simulink model "ADU_Integration_Y2016_simulation"  (R2016b)
settings: Solver=FixedStepDiscrete  StartTime=240  StopTime=300  FixedStep=0.01  RelTol=1e-3  EnableMultiTasking=on
PostLoadFcn:
  | , if any(exist('dsrtsu_mdlpostloadfcn', 'file') == [2, 3, 6]), try dsrtsu_mdlpostloadfcn('Execute', bdroot); catch fprintf('Error in PostLoadFcn (dsrtsu_mdlpostloadfcn) for model "%s":\n %s\n', bdroot, lasterr); end, end,
InitFcn:
  | load 'data/chi2_dat';
  | load 'data/innerLine_struct';
  | load 'data/middleLine_struct';
  | load 'data/outerLine_struct';
  | load 'data/innerLine';
  | load 'data/middleLine';
  | load 'data/outerLine';
  | load 'data/landmarks_patac_schimmel_ccw';
  | load 'data/patac_navi_array';
  | load 'data/sensor';
  | load 'data/map_struct';
  | addpath map_src
  | Integration_Parameter;
  | load 'TestData_001';
values from neighbouring files (symbols this model uses):
  TestData_001 =     [TestData_001.mat]
undefined symbols (not defined in the file or in its folder): a, chi2_dat, innerLine, landmarks_patac_schimmel_ccw, middleLine, outerLine, patac_navi_array, StartNum
libraries: simulink x36, rtican x1
(part 7 of 20)

== system ADU_Integration_Y2016_simulation/LogData/Vision_Target/EPM_Lane_Signals ==
  1-D Lookup Table1 : Lookup_n-D  NumberOfTableDimensions=1  BreakpointsForDimension1=TestData_001.X.Data  Table=TestData_001.Y(667).Data  RndMeth=Simplest  InputSameDT=on
  1-D Lookup Table10 : Lookup_n-D  NumberOfTableDimensions=1  BreakpointsForDimension1=TestData_001.X.Data  Table=TestData_001.Y(687).Data  RndMeth=Simplest  InputSameDT=on
  1-D Lookup Table11 : Lookup_n-D  NumberOfTableDimensions=1  BreakpointsForDimension1=TestData_001.X.Data  Table=TestData_001.Y(688).Data  RndMeth=Simplest  InputSameDT=on
  1-D Lookup Table12 : Lookup_n-D  NumberOfTableDimensions=1  BreakpointsForDimension1=TestData_001.X.Data  Table=TestData_001.Y(689).Data  RndMeth=Simplest  InputSameDT=on
  1-D Lookup Table13 : Lookup_n-D  NumberOfTableDimensions=1  BreakpointsForDimension1=TestData_001.X.Data  Table=TestData_001.Y(692).Data  RndMeth=Simplest  InputSameDT=on
  1-D Lookup Table14 : Lookup_n-D  NumberOfTableDimensions=1  BreakpointsForDimension1=TestData_001.X.Data  Table=TestData_001.Y(694).Data  RndMeth=Simplest  InputSameDT=on
  1-D Lookup Table15 : Lookup_n-D  NumberOfTableDimensions=1  BreakpointsForDimension1=TestData_001.X.Data  Table=TestData_001.Y(695).Data  RndMeth=Simplest  InputSameDT=on
  1-D Lookup Table190 : Lookup_n-D  NumberOfTableDimensions=1  BreakpointsForDimension1=TestData_001.X.Data  Table=TestData_001.Y(666).Data  RndMeth=Simplest  InputSameDT=on
  1-D Lookup Table2 : Lookup_n-D  NumberOfTableDimensions=1  BreakpointsForDimension1=TestData_001.X.Data  Table=TestData_001.Y(663).Data  RndMeth=Simplest  InputSameDT=on
  1-D Lookup Table3 : Lookup_n-D  NumberOfTableDimensions=1  BreakpointsForDimension1=TestData_001.X.Data  Table=TestData_001.Y(664).Data  RndMeth=Simplest  InputSameDT=on
  1-D Lookup Table4 : Lookup_n-D  NumberOfTableDimensions=1  BreakpointsForDimension1=TestData_001.X.Data  Table=TestData_001.Y(665).Data  RndMeth=Simplest  InputSameDT=on
  1-D Lookup Table5 : Lookup_n-D  NumberOfTableDimensions=1  BreakpointsForDimension1=TestData_001.X.Data  Table=TestData_001.Y(668).Data  RndMeth=Simplest  InputSameDT=on
  1-D Lookup Table6 : Lookup_n-D  NumberOfTableDimensions=1  BreakpointsForDimension1=TestData_001.X.Data  Table=TestData_001.Y(670).Data  RndMeth=Simplest  InputSameDT=on
  1-D Lookup Table7 : Lookup_n-D  NumberOfTableDimensions=1  BreakpointsForDimension1=TestData_001.X.Data  Table=TestData_001.Y(671).Data  RndMeth=Simplest  InputSameDT=on
  1-D Lookup Table8 : Lookup_n-D  NumberOfTableDimensions=1  BreakpointsForDimension1=TestData_001.X.Data  Table=TestData_001.Y(690).Data  RndMeth=Simplest  InputSameDT=on
  1-D Lookup Table9 : Lookup_n-D  NumberOfTableDimensions=1  BreakpointsForDimension1=TestData_001.X.Data  Table=TestData_001.Y(691).Data  RndMeth=Simplest  InputSameDT=on
  Bus Creator{,3,5,7} (4 alike) : BusCreator  Inputs=7
  Bus Creator1 : BusCreator  Inputs=19
  Bus Creator2 : BusCreator  Inputs=8
  Bus Creator4 : BusCreator  Inputs=19
  Bus Creator6 : BusCreator  Inputs=6
  Bus Creator8 : BusCreator  Inputs=6
  EPM_Lane_Singals : Outport
  wires:
  Bus Creator/1 -> Bus Creator2/1  "LKA_Left_Lane_A"
  ? -> Bus Creator3/7  "Rx_Time"
  Bus Creator2/1 -> EPM_Lane_Singals/1  "EPM_Lane_BUS"
  Bus Creator3/1 -> Bus Creator2/3  "LKA_Right_Lane_A"
  1-D Lookup Table8/1 -> Bus Creator3/1  "Lane_Type"
  1-D Lookup Table9/1 -> Bus Creator3/2  "Quality"
  Bus Creator4/1 -> Bus Creator2/4  "LKA_Right_Lane_B"
  Bus Creator1/1 -> Bus Creator2/2  "LKA_Left_Lane_B"
  1-D Lookup Table1/1 -> Bus Creator/2  "Quality"
  1-D Lookup Table190/1 -> Bus Creator/1  "Lane_Type"
  ? -> Bus Creator5/2  "Quality"
  ? -> Bus Creator5/1  "Lane_Type"
  ? -> Bus Creator5/7  "Rx_Time"
  ? -> Bus Creator7/2  "Quality"
  ? -> Bus Creator7/1  "Lane_Type"
  ? -> Bus Creator7/7  "Rx_Time"
  Bus Creator8/1 -> Bus Creator2/8  "Next_Right_Lane_B"
  Bus Creator7/1 -> Bus Creator2/7  "Next_Right_Lane_A"
  Bus Creator5/1 -> Bus Creator2/5  "Next_Left_Lane_A"
  Bus Creator6/1 -> Bus Creator2/6  "Next_Left_Lane_B"
  1-D Lookup Table4/1 -> Bus Creator/5  "Lane_Model_C3"
  1-D Lookup Table2/1 -> Bus Creator/3  "Lane_Model_C0"
  1-D Lookup Table5/1 -> Bus Creator/6  "Width_marking"
  1-D Lookup Table3/1 -> Bus Creator/4  "Lane_Model_C2"
  1-D Lookup Table6/1 -> Bus Creator1/1  "Lane_Model_C1"
  ? -> Bus Creator1/4  "reserved2_laneB"
  ? -> Bus Creator1/18  "TLC"
  ? -> Bus Creator1/9  "PRED_OVERRIDE"
  ? -> Bus Creator1/12  "Reserved1_laneB"
  ? -> Bus Creator1/2  "View_Range_Start"
  ? -> Bus Creator1/16  "PRED_SOURCE_STD"
  ? -> Bus Creator1/15  "PRED_SOURCE_HWE_SPAIN"
  ? -> Bus Creator1/5  "Lane_Crossing"
  1-D Lookup Table7/1 -> Bus Creator1/6  "Lane_mark_color"
  ? -> Bus Creator1/7  "PRED_DIST_BASED_EXTRAPOLATION"
  ? -> Bus Creator1/10  "PRED_OCCLUDED_LM_EXTRAPOLATION"
  ? -> Bus Creator1/11  "PRED_HEADWAY_ORIENTED"
  ? -> Bus Creator1/13  "PRED_SOURCE_DIVERGING_LANES"
  ? -> Bus Creator1/14  "PRED_SOURCE_GUARDRAIL_SHADOW"
  ? -> Bus Creator1/17  "PRED_SOURCE_VRTL_MERGE"
  ? -> Bus Creator1/19  "Rx_Time"
  ? -> Bus Creator1/3  "View_Range_End"
  ? -> Bus Creator1/8  "PRED_OTHER_SIDE"
  1-D Lookup Table12/1 -> Bus Creator3/5  "Lane_Model_C3"
  1-D Lookup Table13/1 -> Bus Creator3/6  "Width_marking"
  1-D Lookup Table10/1 -> Bus Creator3/3  "Lane_Model_C0"
  1-D Lookup Table11/1 -> Bus Creator3/4  "Lane_Model_C2"
  1-D Lookup Table14/1 -> Bus Creator4/1  "Lane_Model_C1"
  ? -> Bus Creator4/3  "View_Range_End"
  ? -> Bus Creator4/10  "PRED_OCCLUDED_LM_EXTRAPOLATION"
  ? -> Bus Creator4/12  "Reserved1_laneB"
  ? -> Bus Creator4/14  "PRED_SOURCE_GUARDRAIL_SHADOW"
  ? -> Bus Creator4/2  "View_Range_Start"
  ? -> Bus Creator4/5  "Lane_Crossing"
  1-D Lookup Table15/1 -> Bus Creator4/6  "Lane_mark_color"
  ? -> Bus Creator4/7  "PRED_DIST_BASED_EXTRAPOLATION"
  ? -> Bus Creator4/8  "PRED_OTHER_SIDE"
  ? -> Bus Creator4/11  "PRED_HEADWAY_ORIENTED"
  ? -> Bus Creator4/13  "PRED_SOURCE_DIVERGING_LANES"
  ? -> Bus Creator4/15  "PRED_SOURCE_HWE_SPAIN"
  ? -> Bus Creator4/9  "PRED_OVERRIDE"
  ? -> Bus Creator4/16  "PRED_SOURCE_STD"
  ? -> Bus Creator4/17  "PRED_SOURCE_VRTL_MERGE"
  ? -> Bus Creator4/18  "TLC"
  ? -> Bus Creator4/19  "Rx_Time"
  ? -> Bus Creator4/4  "reserved2_laneB"
  ? -> Bus Creator5/6  "Width_marking"
  ? -> Bus Creator5/4  "Lane_Model_C2"
  ? -> Bus Creator5/3  "Lane_Model_C0"
  ? -> Bus Creator5/5  "Lane_Model_C3"
  ? -> Bus Creator6/1  "Lane_Model_C1"
  ? -> Bus Creator6/2  "View_Range_Start"
  ? -> Bus Creator6/3  "View_Range_End"
  ? -> Bus Creator6/4  "Lane_mark_color"
  ? -> Bus Creator6/5  "reserved_bits5"
  ? -> Bus Creator6/6  "Rx_Time"
  ? -> Bus Creator7/5  "Lane_Model_C3"
  ? -> Bus Creator7/4  "Lane_Model_C2"
  ? -> Bus Creator7/3  "Lane_Model_C0"
  ? -> Bus Creator7/6  "Width_marking"
  ? -> Bus Creator8/4  "Lane_mark_color"
  ? -> Bus Creator8/5  "reserved_bits5"
  ? -> Bus Creator8/1  "Lane_Model_C1"
  ? -> Bus Creator8/2  "View_Range_Start"
  ? -> Bus Creator8/3  "View_Range_End"
  ? -> Bus Creator8/6  "Rx_Time"
  [Clock] -> 1-D Lookup Table1/1, 1-D Lookup Table3/1, 1-D Lookup Table4/1, 1-D Lookup Table7/1, 1-D Lookup Table6/1, 1-D Lookup Table5/1, 1-D Lookup Table2/1, 1-D Lookup Table190/1
  [Clock] -> 1-D Lookup Table13/1, 1-D Lookup Table15/1, 1-D Lookup Table14/1, 1-D Lookup Table12/1, 1-D Lookup Table11/1, 1-D Lookup Table10/1, 1-D Lookup Table9/1, 1-D Lookup Table8/1

== system ADU_Integration_Y2016_simulation/Path_Plan1/InterSectionPathPlanningModule/PathCreater ==
  RoadInfo : Inport
  ObjInfo : Inport  Port=2
  TrigFlg : Inport  Port=3
  2-D Lookup Table : Lookup_n-D  BreakpointsForDimension1=[0 50]  BreakpointsForDimension2=[0 0.2]  Table=[1 1;1 1]  InternalRulePriority=Speed  RndMeth=Simplest  InputSameDT=on
  Bus Creator2 : BusCreator  Inputs=7
  Bus Selector : BusSelector  OutputSignals=x_in,y_in,angle_in,x_out,y_out,angle_out
  Bus Selector2 : BusSelector  OutputSignals=Info_Ld,Info_Fd,Info_Me
  Demux : Demux  Outputs=5
  MATLAB Function : MATLAB Function  TreatAsAtomicUnit=on
  PathInfo : Outport
  PreViewTime : Outport  Port=2
  wires:
  2-D Lookup Table/1 -> PreViewTime/1
  Demux/3 -> 2-D Lookup Table/1
  TrigFlg/1 -> MATLAB Function/10(TrigFlg)
  RoadInfo/1 -> Bus Selector/1
  Bus Creator2/1 -> PathInfo/1
  MATLAB Function/1(xoptres) -> Bus Creator2/1  "xoptres"
  MATLAB Function/3(Arclengthout) -> Bus Creator2/3  "Arclengthout"
  MATLAB Function/5(T_lat) -> Bus Creator2/5  "T_lat"
  MATLAB Function/4(T_long) -> Bus Creator2/4  "T_long"
  MATLAB Function/7(KurMax) -> Bus Creator2/7, 2-D Lookup Table/2  "KurMax"
  MATLAB Function/2(Deltaout) -> Bus Creator2/2  "Deltaout"
  MATLAB Function/6(PlanRes) -> Bus Creator2/6  "PlanRes"
  ObjInfo/1 -> Bus Selector2/1
  Bus Selector2/3 -> MATLAB Function/9(Info_Me), Demux/1  "<Info_Me>"
  Bus Selector2/2 -> MATLAB Function/8(Info_Fd)  "<Info_Fd>"
  Bus Selector/5 -> MATLAB Function/5(y_out)  "<y_out>"
  Bus Selector/3 -> MATLAB Function/3(angle_in)  "<angle_in>"
  Bus Selector/1 -> MATLAB Function/1(x_in)  "<x_in>"
  Bus Selector/6 -> MATLAB Function/6(angle_out)  "<angle_out>"
  Bus Selector2/1 -> MATLAB Function/7(Info_Ld)  "<Info_Ld>"
  Bus Selector/4 -> MATLAB Function/4(x_out)  "<x_out>"
  Bus Selector/2 -> MATLAB Function/2(y_in)  "<y_in>"

== system ADU_Integration_Y2016_simulation/Path_Plan1/InterSectionPathPlanningModule/PathPrePointCal ==
  RoadInfo : Inport
  PathInfo : Inport  Port=2
  PreTime : Inport  Port=3
  VehicleInfo : Inport  Port=4
  Bus Creator2 : BusCreator  Inputs=7
  Bus Selector1 : BusSelector  OutputSignals=x_in,y_in,angle_in,x_out,y_out,angle_out
  Bus Selector3 : BusSelector  OutputSignals=xoptres,Deltaout,Arclengthout,T_long,T_lat,PlanRes,KurMax
  PrePointCal : MATLAB Function  TreatAsAtomicUnit=on
  Terminator13 : Terminator
  PathPlanningSuccessFlg : Outport
  PrePointInfo : Outport  Port=2
  PathTrigFinishFlg : Outport  Port=3
  wires:
  PrePointCal/8(PathTrjFinishFlg) -> PathTrigFinishFlg/1
  PreTime/1 -> PrePointCal/13(Time)
  PathInfo/1 -> Bus Selector3/1
  Bus Selector3/7 -> Terminator13/1  "<KurMax>"
  Bus Selector3/2 -> PrePointCal/2(Delta)  "<Deltaout>"
  Bus Selector3/5 -> PrePointCal/5(T_lat)  "<T_lat>"
  Bus Selector3/4 -> PrePointCal/4(T_long)  "<T_long>"
  Bus Selector3/6 -> PathPlanningSuccessFlg/1, PrePointCal/14(PathPlanRes)  "<PlanRes>"
  Bus Creator2/1 -> PrePointInfo/1
  Bus Selector3/1 -> PrePointCal/1(V_tar)  "<xoptres>"
  Bus Selector3/3 -> PrePointCal/3(Arclength)  "<Arclengthout>"
  PrePointCal/4(Ay) -> Bus Creator2/4  "Ay"
  PrePointCal/6(Vy) -> Bus Creator2/6  "Vy"
  PrePointCal/7(Theta) -> Bus Creator2/7  "Theta"
  PrePointCal/2(yposition) -> Bus Creator2/2  "yposition"
  PrePointCal/5(Vx) -> Bus Creator2/5  "Vx"
  PrePointCal/1(xposition) -> Bus Creator2/1  "xposition"
  PrePointCal/3(Ax) -> Bus Creator2/3  "Ax"
  RoadInfo/1 -> Bus Selector1/1
  Bus Selector1/4 -> PrePointCal/10(x_out)  "<x_out>"
  Bus Selector1/1 -> PrePointCal/7(x_in)  "<x_in>"
  VehicleInfo/1 -> PrePointCal/6(Info_Me)
  Bus Selector1/2 -> PrePointCal/8(y_in)  "<y_in>"
  Bus Selector1/3 -> PrePointCal/9(angle_in)  "<angle_in>"
  Bus Selector1/6 -> PrePointCal/12(angle_out)  "<angle_out>"
  Bus Selector1/5 -> PrePointCal/11(y_out)  "<y_out>"

== system ADU_Integration_Y2016_simulation/Path_Plan1/InterSectionPathPlanningModule/PrePointCorConvert ==
  PrePointInfo : Inport
  PathTrjFinishFlg : Inport  Port=2
  LoCorInfo : Inport  Port=3
  Bus Selector1 : BusSelector  OutputSignals=XposLoCur,YposLoCur,ThetaLoCur
  Bus Selector2 : BusSelector  OutputSignals=xposition,yposition,Ax,Ay,Vx,Vy,Theta
  CordConvter : MATLAB Function  TreatAsAtomicUnit=on
  Delay : Delay  DelayLength=1  InitialCondition=0
  Delay1 : Delay  DelayLength=1  InitialCondition=0
  Terminator : Terminator
  Position : Outport
  Motion : Outport  Port=2
  ThetaLo : Outport  Port=3
  wires:
  PathTrjFinishFlg/1 -> Terminator/1
  Delay/1 -> CordConvter/2(xpositionPre)
  Delay1/1 -> CordConvter/4(ypositionPre)
  CordConvter/1(VsPathPlan_h_position) -> Position/1
  CordConvter/2(VsPathPlan_h_Motion) -> Motion/1
  CordConvter/3(ThetaLo) -> ThetaLo/1
  LoCorInfo/1 -> Bus Selector1/1
  Bus Selector1/3 -> CordConvter/12(thetaCur)  "<ThetaLoCur>"
  Bus Selector1/1 -> CordConvter/10(xpositionCur)  "<XposLoCur>"
  Bus Selector1/2 -> CordConvter/11(ypositionCur)  "<YposLoCur>"
  PrePointInfo/1 -> Bus Selector2/1
  Bus Selector2/1 -> Delay/1, CordConvter/1(xpositionTar)  "<xposition>"
  Bus Selector2/4 -> CordConvter/6(Ay)  "<Ay>"
  Bus Selector2/2 -> Delay1/1, CordConvter/3(ypositionTar)  "<yposition>"
  Bus Selector2/3 -> CordConvter/5(Ax)  "<Ax>"
  Bus Selector2/7 -> CordConvter/9(ThetaTar)  "<Theta>"
  Bus Selector2/5 -> CordConvter/7(Vx)  "<Vx>"
  Bus Selector2/6 -> CordConvter/8(Vy)  "<Vy>"

== system ADU_Integration_Y2016_simulation/Path_Plan1/LaneChangePathPlanningModule1/PathCreator ==
  ObjInfo : Inport
  RoadInfo : Inport  Port=2
  VehicleInfo : Inport  Port=3
  TrigFlg : Inport  Port=4
  LongDisLimit : Inport  Port=5
  2-D Lookup Table : Lookup_n-D  BreakpointsForDimension1=[0 50]  BreakpointsForDimension2=[0 0.2]  Table=[1 1;1 1]  InternalRulePriority=Speed  RndMeth=Simplest  InputSameDT=on
  Bus Creator : BusCreator  Inputs=3
  Bus Selector : BusSelector  OutputSignals=Info_Fd,Info_Fo,Info_Ld,Info_Lo
  Bus Selector1 : BusSelector  OutputSignals=x_in,y_in,angle_in,y_out,angle_out
  Constant : Constant  Value=100
  Constant1 : Constant  Value=100
  Demux : Demux  Outputs=5
  PathCreator : MATLAB Function  TreatAsAtomicUnit=on
  PathInfo : Outport
  PreViewTime : Outport  Port=2
  wires:
  Constant1/1 -> PathCreator/14(N2)
  TrigFlg/1 -> PathCreator/11(TrigFlg)
  Constant/1 -> PathCreator/13(N)
  2-D Lookup Table/1 -> PreViewTime/1
  Demux/3 -> 2-D Lookup Table/1
  Bus Creator/1 -> PathInfo/1
  PathCreator/1(xoptres) -> Bus Creator/1  "xoptres"
  Bus Selector/1 -> PathCreator/1(Info_FdIn)  "<Info_Fd>"
  Bus Selector1/2 -> PathCreator/7(y_inIn)  "<y_in>"
  Bus Selector/2 -> PathCreator/2(Info_FoIn)  "<Info_Fo>"
  Bus Selector/3 -> PathCreator/3(Info_LdIn)  "<Info_Ld>"
  RoadInfo/1 -> Bus Selector1/1
  Bus Selector1/1 -> PathCreator/6(x_inIn)  "<x_in>"
  Bus Selector/4 -> PathCreator/4(Info_LoIn)  "<Info_Lo>"
  Bus Selector1/5 -> PathCreator/10(angle_outIn)  "<angle_out>"
  VehicleInfo/1 -> Demux/1, PathCreator/5(Info_MeIn)
  Bus Selector1/4 -> PathCreator/9(y_outIn)  "<y_out>"
  ObjInfo/1 -> Bus Selector/1
  Bus Selector1/3 -> PathCreator/8(angle_inIn)  "<angle_in>"
  PathCreator/3(KurMax) -> 2-D Lookup Table/2, Bus Creator/3  "KurMax"
  PathCreator/2(PlanRes) -> Bus Creator/2  "PlanRes"
  LongDisLimit/1 -> PathCreator/12(X_melimit_In)

== system ADU_Integration_Y2016_simulation/Path_Plan1/LaneChangePathPlanningModule1/PathPrePointCal ==
  PathInfo : Inport
  PreTime : Inport  Port=2
  RoadInfo : Inport  Port=3
  VehicleInfo : Inport  Port=4
  Bus Creator2 : BusCreator  Inputs=7
  Bus Selector1 : BusSelector  OutputSignals=xoptres,PlanRes,KurMax
  Bus Selector2 : BusSelector  OutputSignals=x_in,y_in,angle_in,y_out,angle_out
  PrePointCal : MATLAB Function  TreatAsAtomicUnit=on
  Terminator : Terminator
  PrePointInfo : Outport
  PathTrigFinishFlg : Outport  Port=2
  PathPlanningSuccessFlg : Outport  Port=3
  wires:
  Bus Selector1/3 -> Terminator/1  "<KurMax>"
  Bus Selector1/2 -> PathPlanningSuccessFlg/1  "<PlanRes>"
  Bus Selector1/1 -> PrePointCal/1(xoptres)  "<xoptres>"
  PrePointCal/8(PathTrjFinishFlg) -> PathTrigFinishFlg/1
  PrePointCal/6(Vy) -> Bus Creator2/6  "Vy"
  PrePointCal/3(Ax) -> Bus Creator2/3  "Ax"
  PrePointCal/4(Ay) -> Bus Creator2/4  "Ay"
  PrePointCal/1(xposition) -> Bus Creator2/1  "xposition"
  PrePointCal/2(yposition) -> Bus Creator2/2  "yposition"
  PrePointCal/5(Vx) -> Bus Creator2/5  "Vx"
  PrePointCal/7(Theta) -> Bus Creator2/7  "Theta"
  Bus Creator2/1 -> PrePointInfo/1
  VehicleInfo/1 -> PrePointCal/7(Info_Me)
  RoadInfo/1 -> Bus Selector2/1
  PreTime/1 -> PrePointCal/8(Time)
  Bus Selector2/2 -> PrePointCal/3(y_in)  "<y_in>"
  Bus Selector2/5 -> PrePointCal/6(angle_out)  "<angle_out>"
  Bus Selector2/3 -> PrePointCal/4(angle_in)  "<angle_in>"
  Bus Selector2/1 -> PrePointCal/2(x_in)  "<x_in>"
  Bus Selector2/4 -> PrePointCal/5(y_out)  "<y_out>"
  PathInfo/1 -> Bus Selector1/1

== system ADU_Integration_Y2016_simulation/Path_Plan1/LaneChangePathPlanningModule1/PrePointCorConvert ==
  PrePointInfo : Inport
  PathTrjFinishFlg : Inport  Port=2
  LoCorInfo : Inport  Port=3
  Bus Selector2 : BusSelector  OutputSignals=XposLoCur,YposLoCur,ThetaLoCur
  Bus Selector3 : BusSelector  OutputSignals=xposition,yposition,Ax,Ay,Vx,Vy,Theta
  CordConvert : MATLAB Function  TreatAsAtomicUnit=on
  Delay : Delay  DelayLength=1  InitialCondition=0
  Delay1 : Delay  DelayLength=1  InitialCondition=0
  Terminator : Terminator
  Position : Outport
  Motion : Outport  Port=2
  ThetaLo : Outport  Port=3
  wires:
  PathTrjFinishFlg/1 -> Terminator/1
  Bus Selector3/5 -> CordConvert/7(Vx)  "<Vx>"
  Bus Selector3/7 -> CordConvert/9(ThetaTar)  "<Theta>"
  Bus Selector3/6 -> CordConvert/8(Vy)  "<Vy>"
  Bus Selector3/3 -> CordConvert/5(Ax)  "<Ax>"
  Bus Selector3/1 -> CordConvert/1(xpositionTar), Delay/1  "<xposition>"
  Bus Selector3/2 -> CordConvert/3(ypositionTar), Delay1/1  "<yposition>"
  Bus Selector3/4 -> CordConvert/6(Ay)  "<Ay>"
  CordConvert/3(ThetaLo) -> ThetaLo/1
  CordConvert/2(VsPathPlan_h_Motion) -> Motion/1
  CordConvert/1(VsPathPlan_h_position) -> Position/1
  Delay1/1 -> CordConvert/4(ypositionPre)
  Delay/1 -> CordConvert/2(xpositionPre)
  Bus Selector2/3 -> CordConvert/12(thetaCur)  "<ThetaLoCur>"
  Bus Selector2/2 -> CordConvert/11(ypositionCur)  "<YposLoCur>"
  LoCorInfo/1 -> Bus Selector2/1
  Bus Selector2/1 -> CordConvert/10(xpositionCur)  "<XposLoCur>"
  PrePointInfo/1 -> Bus Selector3/1

== system ADU_Integration_Y2016_simulation/Fusion_Model/Fusion_Block/Global_Fusion/Curve_Radius[m] ==
  Constant : Constant
  Divide : Product  Inputs=*/
  Saturation2 : Saturate  UpperLimit=8191  LowerLimit=0.5
  Curve_Radius[m] : Outport
  wires:
  Constant/1 -> Divide/1
  Saturation2/1 -> Curve_Radius[m]/1
  Divide/1 -> Saturation2/1
  [VehPathCurve] -> Divide/2

== system ADU_Integration_Y2016_simulation/Fusion_Model/Fusion_Block/Global_Fusion/ESR_TemporalAlig/TemporalAligFront ==
  range : Inport
  azimuth : Inport  Port=2
  W : Inport  Port=3  OutDataTypeStr=double  PortDimensions=1
  L : Inport  Port=4  OutDataTypeStr=double  PortDimensions=1
  InstallAngESR : Inport  Port=5  OutDataTypeStr=double  PortDimensions=1
  f : TriggerPort  TriggerType=function-call  VariantControl=Variant
      settings: CopyFcn=Stateflow.SLINSF.SimulinkMan.removeBlockPreDeleteFcn  PreDeleteFcn=Stateflow.SLINSF.SimulinkMan.unsafePredeleteFcn
  Gain1 : Gain  Gain=-1
  Product : Product
  Product1 : Product
  Terminator : Terminator
  Terminator1 : Terminator
  Terminator2 : Terminator
  Trigonometric Function : Trigonometry
  Trigonometric Function1 : Trigonometry  Operator=cos
  rangeX : Outport
  rangeY : Outport  Port=2
  wires:
  L/1 -> Terminator/1
  InstallAngESR/1 -> Terminator1/1
  W/1 -> Terminator2/1
  range/1 -> Product1/1, Product/1  "Range"
  azimuth/1 -> Gain1/1  "Azimuth"
  Trigonometric Function/1 -> Product/2
  Product/1 -> rangeY/1
  Product1/1 -> rangeX/1
  Trigonometric Function1/1 -> Product1/2
  Gain1/1 -> Trigonometric Function1/1, Trigonometric Function/1

== system ADU_Integration_Y2016_simulation/Fusion_Model/Fusion_Block/Global_Fusion/Fusion_Center/FusTrackIni.ESRInPathJudge ==
  x : Inport
  y : Inport  Port=2
  R : Inport  Port=3  OutDataTypeStr=double  PortDimensions=1
  f : TriggerPort  TriggerType=function-call  VariantControl=Variant
      settings: CopyFcn=Stateflow.SLINSF.SimulinkMan.removeBlockPreDeleteFcn  PreDeleteFcn=Stateflow.SLINSF.SimulinkMan.unsafePredeleteFcn
  Abs : Abs
  Compare To Constant : simulink/Logic and Bit Operations/Compare To Constant  relop=<=  const=5  OutDataTypeStr=uint8
  DistanceToRearAxis : Constant  Value=2.6
  Product : Product
  Product1 : Product
  Sqrt1 : Math  Operator=sqrt  OutputSignalType=real  SaturateOnIntegerOverflow=on
  Subtract : Sum
  Subtract1 : Sum  Inputs=+-
  Subtract2 : Sum
  Subtract3 : Sum  Inputs=+-
  InPathFlag : Outport
  wires:
  Product/1 -> Subtract2/1
  x/1 -> Subtract/1  "Range"
  DistanceToRearAxis/1 -> Subtract/2
  Subtract/1 -> Product/2, Product/1
  y/1 -> Subtract1/1  "Azimuth"
  R/1 -> Subtract3/2, Subtract1/2
  Subtract1/1 -> Product1/2, Product1/1
  Product1/1 -> Subtract2/2
  Subtract2/1 -> Sqrt1/1
  Sqrt1/1 -> Subtract3/1
  Compare To Constant/1 -> InPathFlag/1
  Subtract3/1 -> Abs/1
  Abs/1 -> Compare To Constant/1

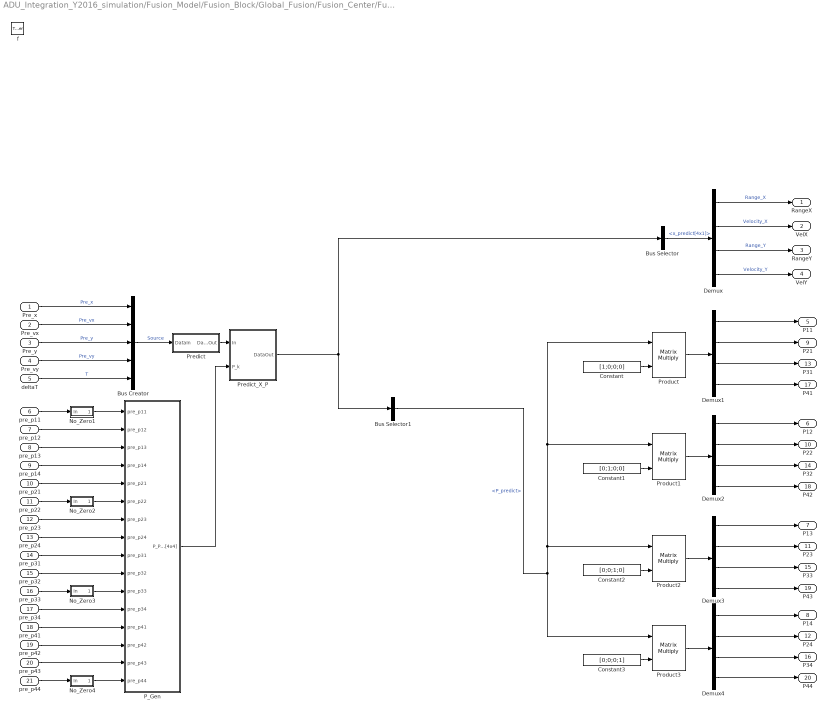
== system ADU_Integration_Y2016_simulation/Fusion_Model/Fusion_Block/Global_Fusion/Fusion_Center/FusTrackPredict.Forecast ==
  Pre_x : Inport
  Pre_vx : Inport  Port=2
  Pre_y : Inport  Port=3
  Pre_vy : Inport  Port=4
  deltaT : Inport  Port=5
  pre_p11 : Inport  Port=6
  pre_p12 : Inport  Port=7
  pre_p13 : Inport  Port=8
  pre_p14 : Inport  Port=9
  pre_p21 : Inport  Port=10
  pre_p22 : Inport  Port=11
  pre_p23 : Inport  Port=12
  pre_p24 : Inport  Port=13
  pre_p31 : Inport  Port=14
  pre_p32 : Inport  Port=15
  pre_p33 : Inport  Port=16
  pre_p34 : Inport  Port=17
  pre_p41 : Inport  Port=18
  pre_p42 : Inport  Port=19
  pre_p43 : Inport  Port=20
  pre_p44 : Inport  Port=21
  f : TriggerPort  TriggerType=function-call  VariantControl=Variant
      settings: CopyFcn=Stateflow.SLINSF.SimulinkMan.removeBlockPreDeleteFcn  PreDeleteFcn=Stateflow.SLINSF.SimulinkMan.unsafePredeleteFcn
  Bus Creator : BusCreator  Inputs=5
  Bus Selector : BusSelector  OutputSignals=x_predict[4x1]
  Bus Selector1 : BusSelector  OutputSignals=P_predict
  Constant : Constant  Value=[1;0;0;0]
  Constant1 : Constant  Value=[0;1;0;0]
  Constant2 : Constant  Value=[0;0;1;0]
  Constant3 : Constant  Value=[0;0;0;1]
  Demux{,1..4} (5 alike) : Demux
  No_Zero1 : Subsystem
  No_Zero2 : Subsystem
  No_Zero3 : Subsystem
  No_Zero4 : Subsystem
  P_Gen : Subsystem
  Predict : Subsystem
  Predict_X_P : Subsystem
  Product{,1..3} (4 alike) : Product  Multiplication=Matrix(*)  RndMeth=Zero
  RangeX : Outport
  VelX : Outport  Port=2
  RangeY : Outport  Port=3
  VelY : Outport  Port=4
  P11 : Outport  Port=5
  P12 : Outport  Port=6
  P13 : Outport  Port=7
  P14 : Outport  Port=8
  P21 : Outport  Port=9
  P22 : Outport  Port=10
  P23 : Outport  Port=11
  P24 : Outport  Port=12
  P31 : Outport  Port=13
  P32 : Outport  Port=14
  P33 : Outport  Port=15
  P34 : Outport  Port=16
  P41 : Outport  Port=17
  P42 : Outport  Port=18
  P43 : Outport  Port=19
  P44 : Outport  Port=20
  wires:
  deltaT/1 -> Bus Creator/5  "T"
  Bus Creator/1 -> Predict/1(DataIn)  "Source"
  Predict/1(DataOut) -> Predict_X_P/1(In)
  Predict_X_P/1(DataOut) -> Bus Selector/1, Bus Selector1/1
  Pre_x/1 -> Bus Creator/1  "Pre_x"
  Pre_vy/1 -> Bus Creator/4  "Pre_vy"
  Pre_y/1 -> Bus Creator/3  "Pre_y"
  Pre_vx/1 -> Bus Creator/2  "Pre_vx"
  P_Gen/1(P_Pre[4x4]) -> Predict_X_P/2(P_k)
  pre_p11/1 -> No_Zero1/1(In)
  pre_p12/1 -> P_Gen/2(pre_p12)
  pre_p13/1 -> P_Gen/3(pre_p13)
  pre_p14/1 -> P_Gen/4(pre_p14)
  pre_p21/1 -> P_Gen/5(pre_p21)
  pre_p22/1 -> No_Zero2/1(In)
  pre_p23/1 -> P_Gen/7(pre_p23)
  pre_p24/1 -> P_Gen/8(pre_p24)
  pre_p31/1 -> P_Gen/9(pre_p31)
  pre_p32/1 -> P_Gen/10(pre_p32)
  pre_p33/1 -> No_Zero3/1(In)
  pre_p34/1 -> P_Gen/12(pre_p34)
  pre_p41/1 -> P_Gen/13(pre_p41)
  pre_p42/1 -> P_Gen/14(pre_p42)
  pre_p43/1 -> P_Gen/15(pre_p43)
  pre_p44/1 -> No_Zero4/1(In)
  Constant/1 -> Product/2
  Product/1 -> Demux1/1
  Demux1/1 -> P11/1
  Demux1/2 -> P21/1
  Demux1/3 -> P31/1
  Bus Selector1/1 -> Product/1, Product1/1, Product2/1, Product3/1  "<P_predict>"
  Demux1/4 -> P41/1
  Constant1/1 -> Product1/2
  Product1/1 -> Demux2/1
  Demux2/1 -> P12/1
  Demux2/2 -> P22/1
  Demux2/3 -> P32/1
  Demux2/4 -> P42/1
  Constant2/1 -> Product2/2
  Product2/1 -> Demux3/1
  Demux3/1 -> P13/1
  Demux3/2 -> P23/1
  Demux3/3 -> P33/1
  Demux3/4 -> P43/1
  Constant3/1 -> Product3/2
  Product3/1 -> Demux4/1
  Demux4/1 -> P14/1
  Demux4/2 -> P24/1
  Demux4/3 -> P34/1
  Demux4/4 -> P44/1
  Bus Selector/1 -> Demux/1  "<x_predict[4x1]>"
  No_Zero1/1(Out) -> P_Gen/1(pre_p11)
  No_Zero2/1(Out) -> P_Gen/6(pre_p22)
  No_Zero3/1(Out) -> P_Gen/11(pre_p33)
  No_Zero4/1(Out) -> P_Gen/16(pre_p44)
  Demux/1 -> RangeX/1  "Range_X"
  Demux/2 -> VelX/1  "Velocity_X"
  Demux/3 -> RangeY/1  "Range_Y"
  Demux/4 -> VelY/1  "Velocity_Y"

== system ADU_Integration_Y2016_simulation/Fusion_Model/Fusion_Block/Global_Fusion/Fusion_Center/FusTrackUpdate.MDCal ==
  MeasureRx : Inport
  MeasureRy : Inport  Port=2
  PredictRx : Inport  Port=3
  PredictRy : Inport  Port=4
  P11 : Inport  Port=5
  P12 : Inport  Port=6
  P13 : Inport  Port=7
  P14 : Inport  Port=8
  P21 : Inport  Port=9
  P22 : Inport  Port=10
  P23 : Inport  Port=11
  P24 : Inport  Port=12
  P31 : Inport  Port=13
  P32 : Inport  Port=14
  P33 : Inport  Port=15
  P34 : Inport  Port=16
  P41 : Inport  Port=17
  P42 : Inport  Port=18
  P43 : Inport  Port=19
  P44 : Inport  Port=20
  R11 : Inport  Port=21
  R12 : Inport  Port=22
  R21 : Inport  Port=23
  R22 : Inport  Port=24
  f : TriggerPort  TriggerType=function-call  VariantControl=Variant
      settings: CopyFcn=Stateflow.SLINSF.SimulinkMan.removeBlockPreDeleteFcn  PreDeleteFcn=Stateflow.SLINSF.SimulinkMan.unsafePredeleteFcn
  Divide : Product  Inputs=*/*  Multiplication=Matrix(*)
  Divide1 : Product  Inputs=***  Multiplication=Matrix(*)
  H : Constant  Value=[1 0 0 0;0 0 1 0]
  Math Function : Math  Operator=transpose  SaturateOnIntegerOverflow=on
  Math Function1 : Math  Operator=transpose  SaturateOnIntegerOverflow=on
  Mux : Mux  Inputs=2
  Mux1 : Mux  Inputs=2
  No_Zero1 : Subsystem
  No_Zero2 : Subsystem
  No_Zero3 : Subsystem
  No_Zero4 : Subsystem
  Subsystem : Subsystem
  Subtract : Sum  Inputs=+-
  Subtract1 : Sum
  W_Gen : Subsystem
  MD : Outport
  wires:
  Mux/1 -> Subtract/1
  Mux1/1 -> Subtract/2
  MeasureRx/1 -> Mux/1
  PredictRx/1 -> Mux1/1
  PredictRy/1 -> Mux1/2
  P11/1 -> No_Zero4/1(In)
  P12/1 -> W_Gen/2(R12)
  P13/1 -> W_Gen/3(R13)
  P14/1 -> W_Gen/4(R14)
  P21/1 -> W_Gen/5(R21)
  P22/1 -> No_Zero1/1(In)
  P23/1 -> W_Gen/7(R23)
  P24/1 -> W_Gen/8(R24)
  P31/1 -> W_Gen/9(R31)
  P32/1 -> W_Gen/10(R32)
  P33/1 -> No_Zero2/1(In)
  P34/1 -> W_Gen/12(R34)
  P41/1 -> W_Gen/13(R41)
  P42/1 -> W_Gen/14(R42)
  P43/1 -> W_Gen/15(R43)
  P44/1 -> No_Zero3/1(In)
  Subtract/1 -> Math Function/1, Divide/3  "[2X1]"
  Math Function/1 -> Divide/1  "[1X2]"
  Divide/1 -> MD/1
  No_Zero4/1(Out) -> W_Gen/1(R11)
  No_Zero1/1(Out) -> W_Gen/6(R22)
  No_Zero2/1(Out) -> W_Gen/11(R33)
  No_Zero3/1(Out) -> W_Gen/16(R44)
  MeasureRy/1 -> Mux/2
  R11/1 -> Subsystem/1(R11)
  R12/1 -> Subsystem/2(R12)
  R21/1 -> Subsystem/3(R21)
  R22/1 -> Subsystem/4(R22)
  W_Gen/1(P_Pre) -> Divide1/2  "[4X4]"
  Subsystem/1(R[2x2]) -> Subtract1/2  "[2X2]"
  H/1 -> Math Function1/1, Divide1/1  "[2X4]"
  Math Function1/1 -> Divide1/3  "2X4"
  Divide1/1 -> Subtract1/1  "[2X2]"
  Subtract1/1 -> Divide/2  "[2X2]"

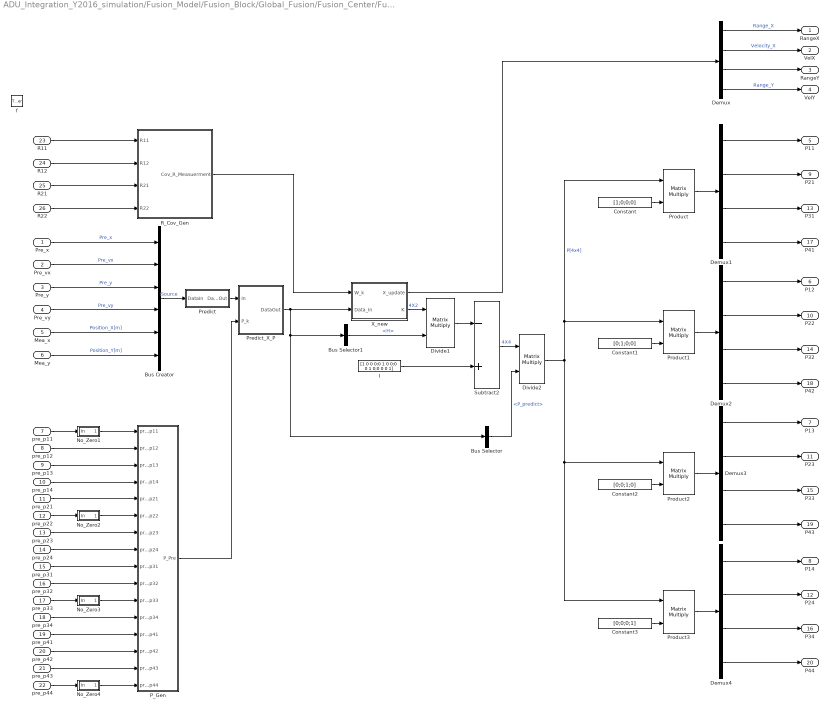
== system ADU_Integration_Y2016_simulation/Fusion_Model/Fusion_Block/Global_Fusion/Fusion_Center/FusTrackUpdate.Update ==
  Pre_x : Inport
  Pre_vx : Inport  Port=2
  Pre_y : Inport  Port=3
  Pre_vy : Inport  Port=4
  Mea_x : Inport  Port=5
  Mea_y : Inport  Port=6
  pre_p11 : Inport  Port=7
  pre_p12 : Inport  Port=8
  pre_p13 : Inport  Port=9
  pre_p14 : Inport  Port=10
  pre_p21 : Inport  Port=11
  pre_p22 : Inport  Port=12
  pre_p23 : Inport  Port=13
  pre_p24 : Inport  Port=14
  pre_p31 : Inport  Port=15
  pre_p32 : Inport  Port=16
  pre_p33 : Inport  Port=17
  pre_p34 : Inport  Port=18
  pre_p41 : Inport  Port=19
  pre_p42 : Inport  Port=20
  pre_p43 : Inport  Port=21
  pre_p44 : Inport  Port=22
  R11 : Inport  Port=23
  R12 : Inport  Port=24
  R21 : Inport  Port=25
  R22 : Inport  Port=26
  f : TriggerPort  TriggerType=function-call  VariantControl=Variant
      settings: CopyFcn=Stateflow.SLINSF.SimulinkMan.removeBlockPreDeleteFcn  PreDeleteFcn=Stateflow.SLINSF.SimulinkMan.unsafePredeleteFcn
  Bus Creator : BusCreator  Inputs=6
  Bus Selector : BusSelector  OutputSignals=P_predict
  Bus Selector1 : BusSelector  OutputSignals=Signal_temp.H
  Constant : Constant  Value=[1;0;0;0]
  Constant1 : Constant  Value=[0;1;0;0]
  Constant2 : Constant  Value=[0;0;1;0]
  Constant3 : Constant  Value=[0;0;0;1]
  Demux{,1..4} (5 alike) : Demux
  Divide1 : Product  Inputs=**  Multiplication=Matrix(*)
  Divide2 : Product  Inputs=**  Multiplication=Matrix(*)
  I : Constant  Value=[1 0 0 0;0 1 0 0;0 0 1 0;0 0 0 1]
  No_Zero1 : Subsystem
  No_Zero2 : Subsystem
  No_Zero3 : Subsystem
  No_Zero4 : Subsystem
  P_Gen : Subsystem
  Predict : Subsystem
  Predict_X_P : Subsystem
  Product{,1..3} (4 alike) : Product  Multiplication=Matrix(*)  RndMeth=Zero
  R_Cov_Gen : Subsystem
  Subtract2 : Sum  Inputs=-+
  X_new : Subsystem
  RangeX : Outport
  VelX : Outport  Port=2
  RangeY : Outport  Port=3
  VelY : Outport  Port=4
  P11 : Outport  Port=5
  P12 : Outport  Port=6
  P13 : Outport  Port=7
  P14 : Outport  Port=8
  P21 : Outport  Port=9
  P22 : Outport  Port=10
  P23 : Outport  Port=11
  P24 : Outport  Port=12
  P31 : Outport  Port=13
  P32 : Outport  Port=14
  P33 : Outport  Port=15
  P34 : Outport  Port=16
  P41 : Outport  Port=17
  P42 : Outport  Port=18
  P43 : Outport  Port=19
  P44 : Outport  Port=20
  wires:
  Mea_x/1 -> Bus Creator/5  "Position_X[m]"
  Mea_y/1 -> Bus Creator/6  "Position_Y[m]"
  Bus Creator/1 -> Predict/1(DataIn)  "Source"
  Predict/1(DataOut) -> Predict_X_P/1(In)
  Predict_X_P/1(DataOut) -> X_new/2(Data_In), Bus Selector/1, Bus Selector1/1
  X_new/2(K) -> Divide1/1  "4X2"
  Bus Selector1/1 -> Divide1/2  "<H>"
  Divide1/1 -> Subtract2/1
  I/1 -> Subtract2/2
  Subtract2/1 -> Divide2/1  "4X4"
  Bus Selector/1 -> Divide2/2  "<P_predict>"
  R_Cov_Gen/1(Cov_R_Measuerment) -> X_new/1(W_k)
  X_new/1(X_update) -> Demux/1
  Pre_x/1 -> Bus Creator/1  "Pre_x"
  Pre_vy/1 -> Bus Creator/4  "Pre_vy"
  Pre_y/1 -> Bus Creator/3  "Pre_y"
  Pre_vx/1 -> Bus Creator/2  "Pre_vx"
  P_Gen/1(P_Pre) -> Predict_X_P/2(P_k)
  pre_p11/1 -> No_Zero1/1(In)
  pre_p12/1 -> P_Gen/2(pre_p12)
  pre_p13/1 -> P_Gen/3(pre_p13)
  pre_p14/1 -> P_Gen/4(pre_p14)
  pre_p21/1 -> P_Gen/5(pre_p21)
  pre_p22/1 -> No_Zero2/1(In)
  pre_p23/1 -> P_Gen/7(pre_p23)
  pre_p24/1 -> P_Gen/8(pre_p24)
  pre_p31/1 -> P_Gen/9(pre_p31)
  pre_p32/1 -> P_Gen/10(pre_p32)
  pre_p33/1 -> No_Zero3/1(In)
  pre_p34/1 -> P_Gen/12(pre_p34)
  pre_p41/1 -> P_Gen/13(pre_p41)
  pre_p42/1 -> P_Gen/14(pre_p42)
  pre_p43/1 -> P_Gen/15(pre_p43)
  pre_p44/1 -> No_Zero4/1(In)
  R11/1 -> R_Cov_Gen/1(R11)
  R12/1 -> R_Cov_Gen/2(R12)
  R21/1 -> R_Cov_Gen/3(R21)
  R22/1 -> R_Cov_Gen/4(R22)
  Constant/1 -> Product/2
  Product/1 -> Demux1/1
  Demux1/1 -> P11/1
  Demux1/2 -> P21/1
  Demux1/3 -> P31/1
  Divide2/1 -> Product3/1, Product2/1, Product/1, Product1/1  "P[4x4]"
  Demux1/4 -> P41/1
  Constant1/1 -> Product1/2
  Product1/1 -> Demux2/1
  Demux2/1 -> P12/1
  Demux2/2 -> P22/1
  Demux2/3 -> P32/1
  Demux2/4 -> P42/1
  Constant2/1 -> Product2/2
  Product2/1 -> Demux3/1
  Demux3/1 -> P13/1
  Demux3/2 -> P23/1
  Demux3/3 -> P33/1
  Demux3/4 -> P43/1
  Constant3/1 -> Product3/2
  Product3/1 -> Demux4/1
  Demux4/1 -> P14/1
  Demux4/2 -> P24/1
  Demux4/3 -> P34/1
  Demux4/4 -> P44/1
  No_Zero1/1(Out) -> P_Gen/1(pre_p11)
  No_Zero2/1(Out) -> P_Gen/6(pre_p22)
  No_Zero3/1(Out) -> P_Gen/11(pre_p33)
  No_Zero4/1(Out) -> P_Gen/16(pre_p44)
  Demux/4 -> VelY/1  "Range_Y"
  Demux/3 -> RangeY/1
  Demux/2 -> VelX/1  "Velocity_X"
  Demux/1 -> RangeX/1  "Range_X"

== system ADU_Integration_Y2016_simulation/Fusion_Model/Fusion_Block/Side_Fusion/LF_SRR_CoordinateAlig/TemporalAligLF ==
  range : Inport
  azimuth : Inport  Port=2
  W : Inport  Port=3  OutDataTypeStr=double  PortDimensions=1
  L : Inport  Port=4  OutDataTypeStr=double  PortDimensions=1
  InstallAngLFSRR : Inport  Port=5  OutDataTypeStr=double  PortDimensions=1
  f : TriggerPort  TriggerType=function-call  VariantControl=Variant
      settings: CopyFcn=Stateflow.SLINSF.SimulinkMan.removeBlockPreDeleteFcn  PreDeleteFcn=Stateflow.SLINSF.SimulinkMan.unsafePredeleteFcn
  Add : Sum  Inputs=-+
  Add1 : Sum
  Add2 : Sum
  Add3 : Sum
  Gain : Gain  Gain=0.5
  LF_SRR_Xoffset[m] : Constant  Value=-0.25
  LF_SRR_Y_offset[m] : Constant  Value=-0.25
  Product : Product
  Product1 : Product
  Terminator : Terminator
  Trigonometric Function : Trigonometry
  Trigonometric Function1 : Trigonometry  Operator=cos
  rangeX : Outport
  rangeY : Outport  Port=2
  wires:
  Trigonometric Function1/1 -> Product1/2
  Product/1 -> Add1/1
  Trigonometric Function/1 -> Product/2
  azimuth/1 -> Add/1  "Azimuth"
  range/1 -> Product/1, Product1/1  "Range"
  W/1 -> Gain/1
  L/1 -> Terminator/1
  InstallAngLFSRR/1 -> Add/2
  Add/1 -> Trigonometric Function1/1, Trigonometric Function/1
  Gain/1 -> Add1/2
  Add1/1 -> Add2/1
  Product1/1 -> Add3/1
  LF_SRR_Y_offset[m]/1 -> Add2/2
  LF_SRR_Xoffset[m]/1 -> Add3/2
  Add2/1 -> rangeY/1
  Add3/1 -> rangeX/1

== system ADU_Integration_Y2016_simulation/Fusion_Model/Fusion_Block/Side_Fusion/LR_SRR_CoordinateAlig/TemporalAligLR ==
  range : Inport
  azimuth : Inport  Port=2
  W : Inport  Port=3  OutDataTypeStr=double  PortDimensions=1
  L : Inport  Port=4  OutDataTypeStr=double  PortDimensions=1
  InstallAngLRSRR : Inport  Port=5  OutDataTypeStr=double  PortDimensions=1
  f : TriggerPort  TriggerType=function-call  VariantControl=Variant
      settings: CopyFcn=Stateflow.SLINSF.SimulinkMan.removeBlockPreDeleteFcn  PreDeleteFcn=Stateflow.SLINSF.SimulinkMan.unsafePredeleteFcn
  Add : Sum
  Add1 : Sum
  Add2 : Sum  Inputs=--
  Gain : Gain  Gain=0.5
  Product : Product
  Product1 : Product
  Trigonometric Function : Trigonometry
  Trigonometric Function1 : Trigonometry  Operator=cos
  rangeX : Outport
  rangeY : Outport  Port=2
  wires:
  Trigonometric Function1/1 -> Product1/2
  Product1/1 -> Add2/2
  Product/1 -> Add1/1
  Trigonometric Function/1 -> Product/2
  azimuth/1 -> Add/1  "Azimuth"
  range/1 -> Product/1, Product1/1  "Range"
  W/1 -> Gain/1
  L/1 -> Add2/1
  InstallAngLRSRR/1 -> Add/2
  Add/1 -> Trigonometric Function1/1, Trigonometric Function/1
  Add1/1 -> rangeY/1
  Gain/1 -> Add1/2
  Add2/1 -> rangeX/1

== system ADU_Integration_Y2016_simulation/Fusion_Model/Fusion_Block/Side_Fusion/RF_SRR_CoordinateAlig/TemporalAligRF ==
  range : Inport
  azimuth : Inport  Port=2
  W : Inport  Port=3  OutDataTypeStr=double  PortDimensions=1
  L : Inport  Port=4  OutDataTypeStr=double  PortDimensions=1
  InstallAngRFSRR : Inport  Port=5  OutDataTypeStr=double  PortDimensions=1
  f : TriggerPort  TriggerType=function-call  VariantControl=Variant
      settings: CopyFcn=Stateflow.SLINSF.SimulinkMan.removeBlockPreDeleteFcn  PreDeleteFcn=Stateflow.SLINSF.SimulinkMan.unsafePredeleteFcn
  Add : Sum  Inputs=-+
  Add1 : Sum  Inputs=--
  Add2 : Sum
  Add3 : Sum
  Gain : Gain  Gain=0.5
  Product : Product
  Product1 : Product
  RF_SRR_Xoffset[m] : Constant  Value=-0.25
  RF_SRR_Y_offset[m] : Constant  Value=0.25
  Terminator : Terminator
  Trigonometric Function : Trigonometry
  Trigonometric Function1 : Trigonometry  Operator=cos
  rangeX : Outport
  rangeY : Outport  Port=2
  wires:
  Gain/1 -> Add1/2
  Add1/1 -> Add2/1
  Add/1 -> Trigonometric Function/1, Trigonometric Function1/1
  InstallAngRFSRR/1 -> Add/2
  L/1 -> Terminator/1
  W/1 -> Gain/1
  range/1 -> Product1/1, Product/1  "Range"
  azimuth/1 -> Add/1  "Azimuth"
  Trigonometric Function/1 -> Product/2
  Product/1 -> Add1/1
  Product1/1 -> Add3/1
  Trigonometric Function1/1 -> Product1/2
  Add2/1 -> rangeY/1
  RF_SRR_Y_offset[m]/1 -> Add2/2
  Add3/1 -> rangeX/1
  RF_SRR_Xoffset[m]/1 -> Add3/2

== system ADU_Integration_Y2016_simulation/Fusion_Model/Fusion_Block/Side_Fusion/RR_SRR_CoordinateAlig/TemporalAligRR ==
  range : Inport
  azimuth : Inport  Port=2
  W : Inport  Port=3  OutDataTypeStr=double  PortDimensions=1
  L : Inport  Port=4  OutDataTypeStr=double  PortDimensions=1
  InstallAngRRSRR : Inport  Port=5  OutDataTypeStr=double  PortDimensions=1
  f : TriggerPort  TriggerType=function-call  VariantControl=Variant
      settings: CopyFcn=Stateflow.SLINSF.SimulinkMan.removeBlockPreDeleteFcn  PreDeleteFcn=Stateflow.SLINSF.SimulinkMan.unsafePredeleteFcn
  Add : Sum
  Add1 : Sum  Inputs=--
  Add2 : Sum  Inputs=--
  Gain : Gain  Gain=0.5
  Product : Product
  Product1 : Product
  Trigonometric Function : Trigonometry
  Trigonometric Function1 : Trigonometry  Operator=cos
  rangeX : Outport
  rangeY : Outport  Port=2
  wires:
  Add2/1 -> rangeX/1
  Gain/1 -> Add1/2
  Add1/1 -> rangeY/1
  Add/1 -> Trigonometric Function/1, Trigonometric Function1/1
  InstallAngRRSRR/1 -> Add/2
  L/1 -> Add2/1
  W/1 -> Gain/1
  range/1 -> Product1/1, Product/1  "Range"
  azimuth/1 -> Add/1  "Azimuth"
  Trigonometric Function/1 -> Product/2
  Product/1 -> Add1/1
  Product1/1 -> Add2/2
  Trigonometric Function1/1 -> Product1/2

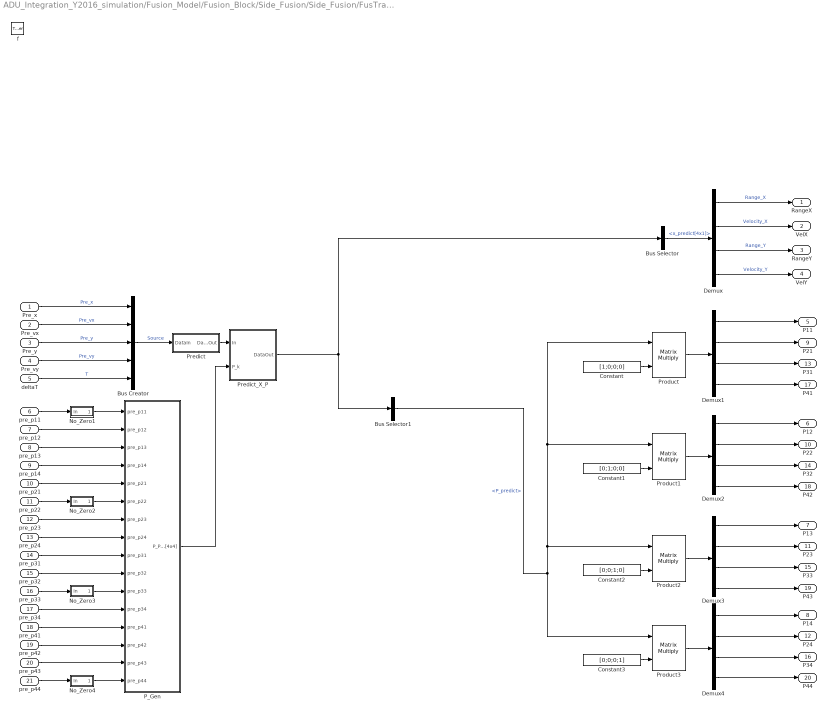
== system ADU_Integration_Y2016_simulation/Fusion_Model/Fusion_Block/Side_Fusion/Side_Fusion/FusTrackPredict.Forecast ==
  Pre_x : Inport
  Pre_vx : Inport  Port=2
  Pre_y : Inport  Port=3
  Pre_vy : Inport  Port=4
  deltaT : Inport  Port=5
  pre_p11 : Inport  Port=6
  pre_p12 : Inport  Port=7
  pre_p13 : Inport  Port=8
  pre_p14 : Inport  Port=9
  pre_p21 : Inport  Port=10
  pre_p22 : Inport  Port=11
  pre_p23 : Inport  Port=12
  pre_p24 : Inport  Port=13
  pre_p31 : Inport  Port=14
  pre_p32 : Inport  Port=15
  pre_p33 : Inport  Port=16
  pre_p34 : Inport  Port=17
  pre_p41 : Inport  Port=18
  pre_p42 : Inport  Port=19
  pre_p43 : Inport  Port=20
  pre_p44 : Inport  Port=21
  f : TriggerPort  TriggerType=function-call  VariantControl=Variant
      settings: CopyFcn=Stateflow.SLINSF.SimulinkMan.removeBlockPreDeleteFcn  PreDeleteFcn=Stateflow.SLINSF.SimulinkMan.unsafePredeleteFcn
  Bus Creator : BusCreator  Inputs=5
  Bus Selector : BusSelector  OutputSignals=x_predict[4x1]
  Bus Selector1 : BusSelector  OutputSignals=P_predict
  Constant : Constant  Value=[1;0;0;0]
  Constant1 : Constant  Value=[0;1;0;0]
  Constant2 : Constant  Value=[0;0;1;0]
  Constant3 : Constant  Value=[0;0;0;1]
  Demux{,1..4} (5 alike) : Demux
  No_Zero1 : Subsystem
  No_Zero2 : Subsystem
  No_Zero3 : Subsystem
  No_Zero4 : Subsystem
  P_Gen : Subsystem
  Predict : Subsystem
  Predict_X_P : Subsystem
  Product{,1..3} (4 alike) : Product  Multiplication=Matrix(*)  RndMeth=Zero
  RangeX : Outport
  VelX : Outport  Port=2
  RangeY : Outport  Port=3
  VelY : Outport  Port=4
  P11 : Outport  Port=5
  P12 : Outport  Port=6
  P13 : Outport  Port=7
  P14 : Outport  Port=8
  P21 : Outport  Port=9
  P22 : Outport  Port=10
  P23 : Outport  Port=11
  P24 : Outport  Port=12
  P31 : Outport  Port=13
  P32 : Outport  Port=14
  P33 : Outport  Port=15
  P34 : Outport  Port=16
  P41 : Outport  Port=17
  P42 : Outport  Port=18
  P43 : Outport  Port=19
  P44 : Outport  Port=20
  wires:
  deltaT/1 -> Bus Creator/5  "T"
  Bus Creator/1 -> Predict/1(DataIn)  "Source"
  Predict/1(DataOut) -> Predict_X_P/1(In)
  Predict_X_P/1(DataOut) -> Bus Selector/1, Bus Selector1/1
  Pre_x/1 -> Bus Creator/1  "Pre_x"
  Pre_vy/1 -> Bus Creator/4  "Pre_vy"
  Pre_y/1 -> Bus Creator/3  "Pre_y"
  Pre_vx/1 -> Bus Creator/2  "Pre_vx"
  P_Gen/1(P_Pre[4x4]) -> Predict_X_P/2(P_k)
  pre_p11/1 -> No_Zero1/1(In)
  pre_p12/1 -> P_Gen/2(pre_p12)
  pre_p13/1 -> P_Gen/3(pre_p13)
  pre_p14/1 -> P_Gen/4(pre_p14)
  pre_p21/1 -> P_Gen/5(pre_p21)
  pre_p22/1 -> No_Zero2/1(In)
  pre_p23/1 -> P_Gen/7(pre_p23)
  pre_p24/1 -> P_Gen/8(pre_p24)
  pre_p31/1 -> P_Gen/9(pre_p31)
  pre_p32/1 -> P_Gen/10(pre_p32)
  pre_p33/1 -> No_Zero3/1(In)
  pre_p34/1 -> P_Gen/12(pre_p34)
  pre_p41/1 -> P_Gen/13(pre_p41)
  pre_p42/1 -> P_Gen/14(pre_p42)
  pre_p43/1 -> P_Gen/15(pre_p43)
  pre_p44/1 -> No_Zero4/1(In)
  Constant/1 -> Product/2
  Product/1 -> Demux1/1
  Demux1/1 -> P11/1
  Demux1/2 -> P21/1
  Demux1/3 -> P31/1
  Bus Selector1/1 -> Product/1, Product1/1, Product2/1, Product3/1  "<P_predict>"
  Demux1/4 -> P41/1
  Constant1/1 -> Product1/2
  Product1/1 -> Demux2/1
  Demux2/1 -> P12/1
  Demux2/2 -> P22/1
  Demux2/3 -> P32/1
  Demux2/4 -> P42/1
  Constant2/1 -> Product2/2
  Product2/1 -> Demux3/1
  Demux3/1 -> P13/1
  Demux3/2 -> P23/1
  Demux3/3 -> P33/1
  Demux3/4 -> P43/1
  Constant3/1 -> Product3/2
  Product3/1 -> Demux4/1
  Demux4/1 -> P14/1
  Demux4/2 -> P24/1
  Demux4/3 -> P34/1
  Demux4/4 -> P44/1
  Bus Selector/1 -> Demux/1  "<x_predict[4x1]>"
  No_Zero1/1(Out) -> P_Gen/1(pre_p11)
  No_Zero2/1(Out) -> P_Gen/6(pre_p22)
  No_Zero3/1(Out) -> P_Gen/11(pre_p33)
  No_Zero4/1(Out) -> P_Gen/16(pre_p44)
  Demux/1 -> RangeX/1  "Range_X"
  Demux/2 -> VelX/1  "Velocity_X"
  Demux/3 -> RangeY/1  "Range_Y"
  Demux/4 -> VelY/1  "Velocity_Y"

== system ADU_Integration_Y2016_simulation/Fusion_Model/Fusion_Block/Side_Fusion/Side_Fusion/G_cal ==
  xt : Inport
  yt : Inport  Port=2
  xj : Inport  Port=3
  yj : Inport  Port=4
  P11 : Inport  Port=5
  P12 : Inport  Port=6
  P13 : Inport  Port=7
  P14 : Inport  Port=8
  P21 : Inport  Port=9
  P22 : Inport  Port=10
  P23 : Inport  Port=11
  P24 : Inport  Port=12
  P31 : Inport  Port=13
  P32 : Inport  Port=14
  P33 : Inport  Port=15
  P34 : Inport  Port=16
  P41 : Inport  Port=17
  P42 : Inport  Port=18
  P43 : Inport  Port=19
  P44 : Inport  Port=20
  R11 : Inport  Port=21
  R12 : Inport  Port=22
  R21 : Inport  Port=23
  R22 : Inport  Port=24
  f : TriggerPort  TriggerType=function-call  VariantControl=Variant
      settings: CopyFcn=Stateflow.SLINSF.SimulinkMan.removeBlockPreDeleteFcn  PreDeleteFcn=Stateflow.SLINSF.SimulinkMan.unsafePredeleteFcn
  Cal_1 : Subsystem
  Divide : Product  Inputs=*/*  Multiplication=Matrix(*)
  Divide1 : Product  Inputs=*/
  Gain : Gain  Gain=-0.5
  H : Constant  Value=[1 0 0 0;0 0 1 0]
  Math Function : Math  Operator=transpose  SaturateOnIntegerOverflow=on
  Math Function1 : Math  SaturateOnIntegerOverflow=on
  Math Function2 : Math  Operator=transpose  SaturateOnIntegerOverflow=on
  Mux1 : Mux  Inputs=2
  Mux2 : Mux  Inputs=2
  No_Zero1 : Subsystem
  No_Zero2 : Subsystem
  No_Zero3 : Subsystem
  No_Zero4 : Subsystem
  No_Zero5 : Subsystem
  No_Zero6 : Subsystem
  P_Gen : Subsystem
  Product : Product  Inputs=3  Multiplication=Matrix(*)  RndMeth=Zero
  Subsystem : Subsystem
  Subtract1 : Sum
  Subtract2 : Sum  Inputs=+-
  Gtj : Outport
  wires:
  No_Zero1/1(Out) -> P_Gen/1(p11)
  No_Zero2/1(Out) -> P_Gen/6(p22)
  No_Zero3/1(Out) -> P_Gen/11(p33)
  No_Zero4/1(Out) -> P_Gen/16(p44)
  Divide1/1 -> Gtj/1  "Gtj"
  P11/1 -> No_Zero1/1(In)
  P12/1 -> P_Gen/2(p12)
  P13/1 -> P_Gen/3(p13)
  P14/1 -> P_Gen/4(p14)
  P21/1 -> P_Gen/5(p21)
  P22/1 -> No_Zero2/1(In)
  P23/1 -> P_Gen/7(p23)
  P32/1 -> P_Gen/10(p32)
  P31/1 -> P_Gen/9(p31)
  P24/1 -> P_Gen/8(p24)
  P33/1 -> No_Zero3/1(In)
  P34/1 -> P_Gen/12(p34)
  P41/1 -> P_Gen/13(p41)
  P42/1 -> P_Gen/14(p42)
  P43/1 -> P_Gen/15(p43)
  P44/1 -> No_Zero4/1(In)
  R11/1 -> No_Zero5/1(In)
  R12/1 -> Subsystem/2(R12)
  R21/1 -> Subsystem/3(R21)
  R22/1 -> No_Zero6/1(In)
  No_Zero5/1(Out) -> Subsystem/1(R11)
  No_Zero6/1(Out) -> Subsystem/4(R22)
  xt/1 -> Mux2/1  "xt"
  yt/1 -> Mux2/2  "yt"
  xj/1 -> Mux1/1  "xj"
  yj/1 -> Mux1/2  "yj"
  Mux2/1 -> Subtract2/1
  Mux1/1 -> Subtract2/2
  Subtract2/1 -> Divide/3, Math Function2/1  "Vtj[2x1]"
  H/1 -> Math Function/1, Product/1  "H[2x4]"
  P_Gen/1(P[4x4]) -> Product/2
  Math Function/1 -> Product/3  "HT[4X2]"
  Product/1 -> Subtract1/1  "2x2"
  Subsystem/1(R[2X2]) -> Subtract1/2  "R[2x2]"
  Subtract1/1 -> Divide/2, Cal_1/1(Stj)  "Stj[2x2]"
  Math Function2/1 -> Divide/1  "Vtj[1x2]"
  Divide/1 -> Gain/1
  Gain/1 -> Math Function1/1
  Math Function1/1 -> Divide1/1
  Cal_1/1(sqrt_det_Stj) -> Divide1/2

== system ADU_Integration_Y2016_simulation/Fusion_Model/Fusion_Block/Side_Fusion/Side_Fusion/Tracker_Initial.VelocityMethod ==
  x_t : Inport
  y_t : Inport  Port=2
  x_m : Inport  Port=3
  y_m : Inport  Port=4
  vx_max : Inport  Port=5
  vx_min : Inport  Port=6
  vy_max : Inport  Port=7
  vy_min : Inport  Port=8
  Rxx : Inport  Port=9
  Ryy : Inport  Port=10
  threshod : Inport  Port=11
  ts : Inport  Port=12
  f : TriggerPort  TriggerType=function-call  VariantControl=Variant
      settings: CopyFcn=Stateflow.SLINSF.SimulinkMan.removeBlockPreDeleteFcn  PreDeleteFcn=Stateflow.SLINSF.SimulinkMan.unsafePredeleteFcn
  Compare To Constant : simulink/Logic and Bit Operations/Compare To Constant  relop=>=  const=0  OutDataTypeStr=uint8
  Constant1 : Constant  Value=0
  Constant2 : Constant  Value=0
  Constant3 : Constant
  Constant4 : Constant  Value=0
  Divide1 : Product  Inputs=***  Multiplication=Matrix(*)
  Dmt : Subsystem
  Math Function1 : Math  Operator=transpose  SaturateOnIntegerOverflow=on
  Multiport Switch : MultiPortSwitch  DataPortOrder=Zero-based contiguous  Inputs=2  zeroidx=on
  R : Subsystem
  Subtract1 : Sum  Inputs=+-
  AssociationFlag : Outport
  wires:
  x_t/1 -> Dmt/1(x_t)
  y_t/1 -> Dmt/2(y_t)
  x_m/1 -> Dmt/3(x_m)
  y_m/1 -> Dmt/4(y_m)
  vx_max/1 -> Dmt/5(vx_max)
  vx_min/1 -> Dmt/6(vx_min)
  vy_max/1 -> Dmt/7(vy_max)
  vy_min/1 -> Dmt/8(vy_min)
  ts/1 -> Dmt/9(ts)
  Ryy/1 -> R/4(R22)
  Rxx/1 -> R/1(R11)
  Constant1/1 -> R/2(R12)
  Constant2/1 -> R/3(R21)
  Dmt/1(dmt[2x1]) -> Divide1/3, Math Function1/1  "[2x1]"
  Math Function1/1 -> Divide1/1  "[1x2]"
  R/1(R[2x2]) -> Divide1/2  "[2x2]]"
  Constant3/1 -> Multiport Switch/2
  Multiport Switch/1 -> AssociationFlag/1
  Divide1/1 -> Subtract1/1
  threshod/1 -> Subtract1/2
  Subtract1/1 -> Compare To Constant/1
  Compare To Constant/1 -> Multiport Switch/1
  Constant4/1 -> Multiport Switch/3

== system ADU_Integration_Y2016_simulation/Fusion_Model/Fusion_Block/Side_Fusion/Side_Fusion/Tracker_Initial.cos_cal ==
  x1 : Inport
  y1 : Inport  Port=2
  x2 : Inport  Port=3
  y2 : Inport  Port=4
  xm : Inport  Port=5
  ym : Inport  Port=6
  f : TriggerPort  TriggerType=function-call  VariantControl=Variant
      settings: CopyFcn=Stateflow.SLINSF.SimulinkMan.removeBlockPreDeleteFcn  PreDeleteFcn=Stateflow.SLINSF.SimulinkMan.unsafePredeleteFcn
  Bus Creator1 : BusCreator  Inputs=6
  Reltive_Deg_Cal : Subsystem
  relative_degree : Outport
  wires:
  x1/1 -> Bus Creator1/1  "x1"
  y1/1 -> Bus Creator1/2  "y1"
  ym/1 -> Bus Creator1/6  "ym"
  xm/1 -> Bus Creator1/5  "xm"
  y2/1 -> Bus Creator1/4  "y2"
  x2/1 -> Bus Creator1/3  "x2"
  Bus Creator1/1 -> Reltive_Deg_Cal/1(In1)
  Reltive_Deg_Cal/1(Rel_Deg) -> relative_degree/1
